simulink model "invPlantAvg_pll"  (R2026a)
settings: Solver=FixedStepDiscrete  StopTime=0.2  FixedStep=ip.Ts_power
model workspace (MATLAB code in the model file):
  | ip = invParams();
libraries: fl_lib x6, nesl_utility x5, ee_lib x4, invLib x2, srfPllLib x1
settings Model: Creator=phamn  LastModifiedBy=aqiba
settings SimscapeCC: SimscapeLogType=none

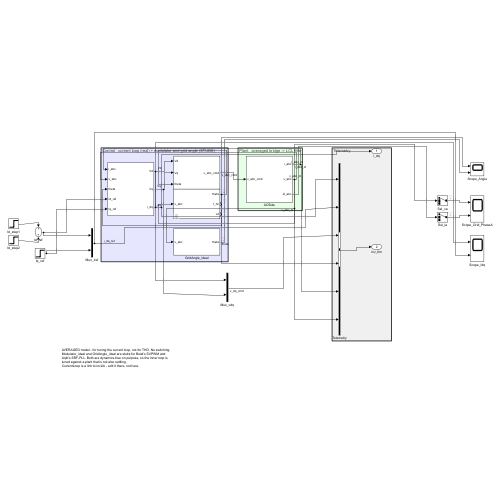
[thumbnail: Simulink's stored preview of the top-level diagram]
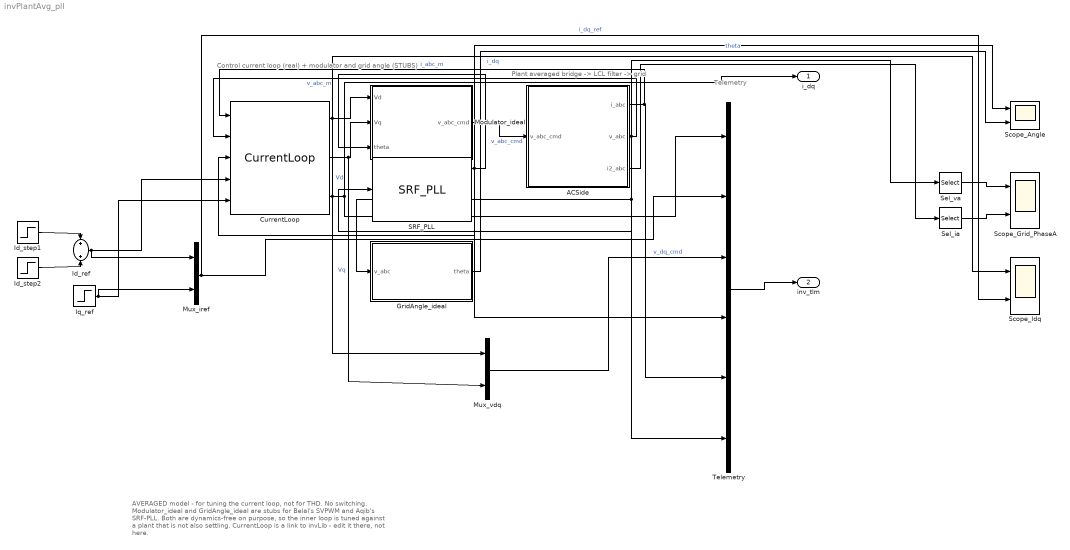
== system invPlantAvg_pll ==
  note: Control current loop (real) + modulator and grid angle (STUBS)
  note: Plant averaged bridge -> LCL filter -> grid
  note: Telemetry
  note: AVERAGED model - for tuning the current loop, not for THD. No switching.
      | Modulator_ideal and GridAngle_ideal are stubs for Belal's SVPWM and
      | Aqib's SRF-PLL. Both are dynamics-free on purpose, so the inner loop is
      | tuned against a plant that is not also settling.
      | CurrentLoop is a link to invLib - edit it there, not here.
  ACSide : Subsystem
  CurrentLoop : invLib/CurrentLoop  SystemSampleTime=-1  VariantActivationTime=update diagram  EmptyChoice=off  PassThrough=off  PassThroughVariantControl=(default)  EmptyChoiceVariantControl=(default)  AllowFlexibleInterface=on  Latency=0  AutoFrameSizeCalculation=off
  GridAngle_ideal : Subsystem
  Id_ref : Sum
  Id_step1 : Step  Time=0.1  FinalValue=0.5*ip.I_pk  SampleTime=0
  Id_step2 : Step  Time=0.13  FinalValue=0.5*ip.I_pk  SampleTime=0
  Iq_ref : Step  Time=0.18  FinalValue=0.25*ip.I_pk  SampleTime=0
  Modulator_ideal : Subsystem
  Mux_iref : Mux  Inputs=2
  Mux_vdq : Mux  Inputs=2
  SRF_PLL : srfPllLib/SRF_PLL  Ts=ip.Ts_ctrl  f0=ip.f_grid  fbw=25  zeta=0.707
  Scope_Angle : Scope  NumInputPorts=2
      settings: SampleTime=1e-5  ActiveDisplayYMinimum=-3.926990816987241  ActiveDisplayYMaximum=3.926990816987241
  Scope_Grid_PhaseA : Scope  NumInputPorts=2
      settings: SampleTime=1e-5  ActiveDisplayYMinimum=-408.248290463863  ActiveDisplayYMaximum=408.248290463863
  Scope_Idq : Scope  NumInputPorts=2
      settings: SampleTime=1e-5  ActiveDisplayYMinimum=-236.06673657757884  ActiveDisplayYMaximum=369.782020323974
  Sel_ia : Selector  InputPortWidth=3  IndexOptions=Index vector (dialog)  Indices=1  OutputSizes=1
  Sel_va : Selector  InputPortWidth=3  IndexOptions=Index vector (dialog)  Indices=1  OutputSizes=1
  Telemetry : BusCreator  Inputs=6
  i_dq : Outport
  inv_tlm : Outport  Port=2
  wires:
  ACSide/1(i_abc) -> CurrentLoop/1, Telemetry/5  "i_abc_m"
  ACSide/2(v_abc) -> GridAngle_ideal/1(v_abc), Telemetry/6, CurrentLoop/2, Sel_va/1, SRF_PLL/1  "v_abc_m"
  CurrentLoop/1 -> Modulator_ideal/1(Vd), Mux_vdq/1  "Vd"
  CurrentLoop/2 -> Modulator_ideal/2(Vq), Mux_vdq/2  "Vq"
  Modulator_ideal/1(v_abc_cmd) -> ACSide/1(v_abc_cmd)  "v_abc_cmd"
  CurrentLoop/3 -> Telemetry/1, i_dq/1, Scope_Idq/1  "i_dq"
  Mux_iref/1 -> Telemetry/2, Scope_Idq/2  "i_dq_ref"
  Mux_vdq/1 -> Telemetry/3  "v_dq_cmd"
  Telemetry/1 -> inv_tlm/1
  Id_step1/1 -> Id_ref/1
  Id_step2/1 -> Id_ref/2
  Id_ref/1 -> CurrentLoop/4, Mux_iref/1
  Iq_ref/1 -> CurrentLoop/5, Mux_iref/2
  ACSide/3(i2_abc) -> Sel_ia/1
  Sel_va/1 -> Scope_Grid_PhaseA/1
  Sel_ia/1 -> Scope_Grid_PhaseA/2
  SRF_PLL/1 -> Modulator_ideal/3(theta), CurrentLoop/3, Telemetry/4, Scope_Angle/1
  GridAngle_ideal/1(theta) -> Scope_Angle/2  "theta"

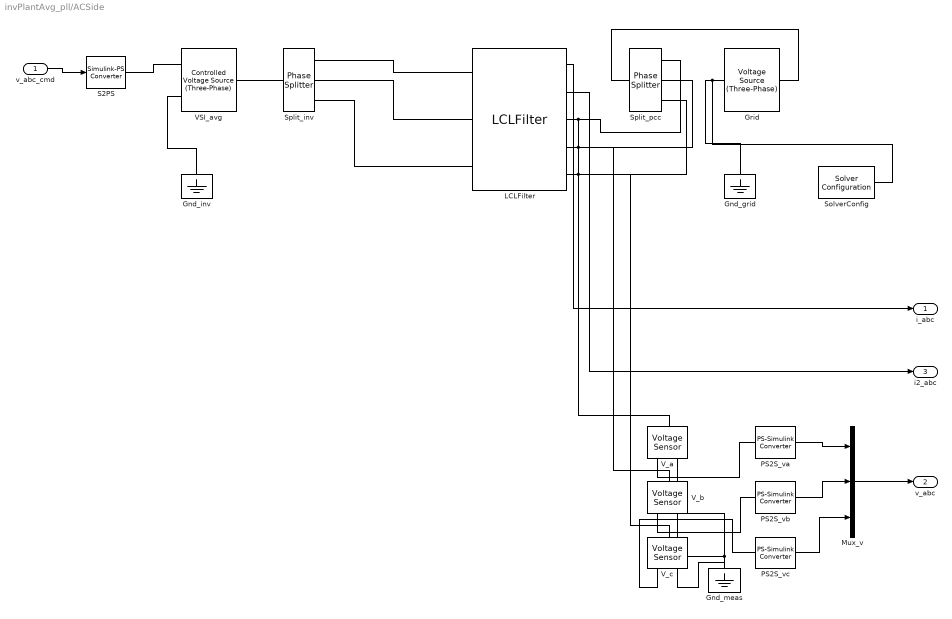
== system invPlantAvg_pll/ACSide ==
  v_abc_cmd : Inport
  Gnd_grid : fl_lib/Electrical/Electrical Elements/Electrical Reference
  Gnd_inv : fl_lib/Electrical/Electrical Elements/Electrical Reference
  Gnd_meas : fl_lib/Electrical/Electrical Elements/Electrical Reference
  Grid : ee_lib/Sources/Voltage Source (Three-Phase)  vline_rms=ip.V_ll V  shift=0 deg  freq=ip.f_grid Hz  impedance_option=ip.grid_Z_opt  SShortCircuit=ip.S_sc A*V  XR=ip.grid_XR  R=0.01 Ohm  L=3.97e-4 H  harmonic_option=1  harmonic_orders=[5, 7]  harmonic_ratios=[0.05, 0.03]  G_parasitic=0 1/Ohm  I_specify=off  I_priority=None  I=[0, 0, 0] A  I_nominal_specify=off  I_nominal_value=1  I_nominal_unit=A
  LCLFilter : invLib/LCLFilter  SystemSampleTime=-1  VariantActivationTime=update diagram  EmptyChoice=off  PassThrough=off  PassThroughVariantControl=(default)  EmptyChoiceVariantControl=(default)  AllowFlexibleInterface=on  Latency=0  AutoFrameSizeCalculation=off
  Mux_v : Mux  Inputs=3
  PS2S_va : nesl_utility/PS-Simulink Converter  PhysicalDomain=network_engine_domain  SubClassName=ps_output  LeftPortType=input  RightPortType=output  PseudoPeriodic=off  Frequencies=[]  VectorFormat=inherit  Unit=inherit  AffineConversion=off
  PS2S_vb : nesl_utility/PS-Simulink Converter  PhysicalDomain=network_engine_domain  SubClassName=ps_output  LeftPortType=input  RightPortType=output  PseudoPeriodic=off  Frequencies=[]  VectorFormat=inherit  Unit=inherit  AffineConversion=off
  PS2S_vc : nesl_utility/PS-Simulink Converter  PhysicalDomain=network_engine_domain  SubClassName=ps_output  LeftPortType=input  RightPortType=output  PseudoPeriodic=off  Frequencies=[]  VectorFormat=inherit  Unit=inherit  AffineConversion=off
  S2PS : nesl_utility/Simulink-PS Converter  PhysicalDomain=network_engine_domain  SubClassName=ps_input  LeftPortType=input  RightPortType=output  PseudoPeriodic=off  Frequencies=[]  NoiseDistribution=none  NoiseParameters=[]  Unit=1  AffineConversion=off  FilteringAndDerivatives=provide  SimscapeFilterOrder=1  InputFilterTimeConstant=0.001  UdotUserProvided=0
  SolverConfig : nesl_utility/Solver Configuration  PhysicalDomain=network_engine_domain  SubClassName=solver  LeftPortType=input  RightPortType=generic  Tones=[]  Harmonics=[]  SimulateNoise=off  Profile=off  UseLocalSampling=off  EnableSwitchedLinearOptims=on  FrequencyDomain=off  UseCCode=off  RelTol=0.001  AbsTol=0.001  MinStep=1e-09  ToWorkspace=off  RevertToSquareIcSolve=off  NumHomotopyIterations=100  PhasorMode=off  PhasorModeNumHarmonics=1  ConsistencySolver=NEWTON_XTOL_AFTER_FTOL  CanonicalOrdering=CANONICAL  OptimizeIntermediates=OPTIMIZED  IndexReductionMethod=DerivativeReplacement  DoDC=off  ResidualTolerance=1e-09  ConsistencyTolSource=GLOBAL  ConsistencyAbsTol=0.001  ConsistencyRelTol=0.001  ConsistencyTolFactor=0.001  UseLocalSolver=on  LocalSolverChoice=NE_BACKWARD_EULER_ADVANCER  ResolveIndetEquations=on  FunctionEvalNumThread=1  LocalSolverSampleTime=ip.Ts_power  DoFixedCost=off  MaxNonlinIter=3  MaxModeIter=2  ComputeImpulses=off  ImpulseIterations=2  LinearAlgebra=auto  LinearAlgebraNumThread=0  EquationFormulation=NE_TIME_EF  DelaysMemoryBudget=1024  AutomaticFiltering=on  FilteringTimeConstant=0.001  PartitionStorageMethod=AS_NEEDED  PartitionMemoryBudget=1024  PartitionMethod=ROBUST  MultibodyUseLocalSolver=off  MultibodyLocalSolverChoice=ODE1  MultibodyLocalSolverSampleTime=0.001
  Split_inv : ee_lib/Connectors & References/Phase Splitter
  Split_pcc : ee_lib/Connectors & References/Phase Splitter
  VSI_avg : ee_lib/Sources/Controlled Voltage Source (Three-Phase)  input_option=ee.enum.inputType.instantaneous  FRated=60 Hz
  V_a : fl_lib/Electrical/Electrical Sensors/Voltage Sensor
  V_b : fl_lib/Electrical/Electrical Sensors/Voltage Sensor
  V_c : fl_lib/Electrical/Electrical Sensors/Voltage Sensor
  i_abc : Outport
  v_abc : Outport  Port=2
  i2_abc : Outport  Port=3
  wires:
  v_abc_cmd/1 -> S2PS/1
  PS2S_va/1 -> Mux_v/1
  PS2S_vb/1 -> Mux_v/2
  PS2S_vc/1 -> Mux_v/3
  LCLFilter/1 -> i_abc/1
  LCLFilter/2 -> i2_abc/1
  Mux_v/1 -> v_abc/1
  connections:
  S2PS/RConn1 -- VSI_avg/LConn1
  Gnd_inv/LConn1 -- VSI_avg/LConn2
  VSI_avg/RConn1 -- Split_inv/LConn1
  Split_pcc/LConn1 -- Grid/RConn1
  Grid/LConn1 -- Gnd_grid/LConn1 -- SolverConfig/RConn1
  Split_inv/RConn1 -- LCLFilter/LConn1
  Split_pcc/RConn1 -- LCLFilter/RConn1 -- V_a/LConn1
  V_a/RConn2 -- V_b/RConn2 -- Gnd_meas/LConn1 -- V_c/RConn2
  V_a/RConn1 -- PS2S_va/LConn1
  Split_inv/RConn2 -- LCLFilter/LConn2
  Split_pcc/RConn2 -- LCLFilter/RConn2 -- V_b/LConn1
  V_b/RConn1 -- PS2S_vb/LConn1
  Split_inv/RConn3 -- LCLFilter/LConn3
  Split_pcc/RConn3 -- LCLFilter/RConn3 -- V_c/LConn1
  V_c/RConn1 -- PS2S_vc/LConn1

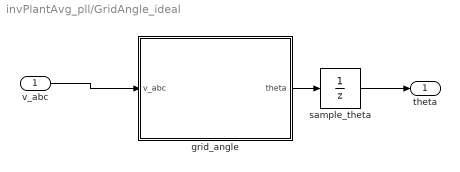
== system invPlantAvg_pll/GridAngle_ideal ==
  v_abc : Inport
  grid_angle : MATLAB Function  TreatAsAtomicUnit=on
  sample_theta : UnitDelay  SampleTime=ip.Ts_ctrl
  theta : Outport
  wires:
  v_abc/1 -> grid_angle/1(v_abc)
  grid_angle/1(theta) -> sample_theta/1
  sample_theta/1 -> theta/1

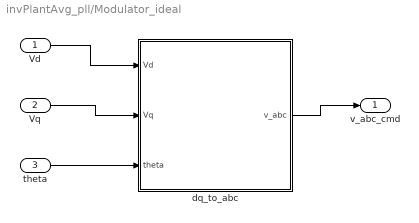
== system invPlantAvg_pll/Modulator_ideal ==
  Vd : Inport
  Vq : Inport  Port=2
  theta : Inport  Port=3
  dq_to_abc : MATLAB Function  TreatAsAtomicUnit=on
  v_abc_cmd : Outport
  wires:
  Vd/1 -> dq_to_abc/1(Vd)
  Vq/1 -> dq_to_abc/2(Vq)
  theta/1 -> dq_to_abc/3(theta)
  dq_to_abc/1(v_abc) -> v_abc_cmd/1

== matlab function invPlantAvg_pll/Modulator_ideal/dq_to_abc ==
  data: Vd input; v_abc output; Vq input; theta input
function v_abc = dq_to_abc(Vd, Vq, theta)
%#codegen
% Inverse of the amplitude-invariant Park transform in invLib/CurrentLoop.
% Stand-in for the modulator: the commanded phase voltages appear directly,
% with no carrier and no V_dc scaling.
v_abc = [ Vd*cos(theta)           - Vq*sin(theta); ...
          Vd*cos(theta - 2*pi/3)  - Vq*sin(theta - 2*pi/3); ...
          Vd*cos(theta + 2*pi/3)  - Vq*sin(theta + 2*pi/3) ];

== matlab function invPlantAvg_pll/GridAngle_ideal/grid_angle ==
  data: v_abc input; theta output
function theta = grid_angle(v_abc)
%#codegen
% Grid voltage angle straight off the Clarke transform. Not a PLL: no loop,
% no filter, no dynamics - which is the point. It gives the inner loop an
% exact angle so the loop can be tuned in isolation, and it gives Aqib's
% SRF-PLL a baseline to be measured against.
v_al = (2/3)*(v_abc(1) - 0.5*v_abc(2) - 0.5*v_abc(3));
v_be = (2/3)*(sqrt(3)/2)*(v_abc(2) - v_abc(3));
theta = atan2(v_be, v_al);
